simulink model "Assignment_model"  (R2015b)
settings: Solver=ode45  StartTime=0.0  StopTime=50  RelTol=1e-3
settings Model: Creator=Administrator  LastModifiedBy=raghavv
settings DataIOCC: SaveFormat=Array
settings DebuggingCC: SolverPrmCheckMsg=warning
settings HardwareCC: ProdBitPerPointer=32  ProdLargestAtomicFloat=None  ProdIntDivRoundTo=Undefined  ProdEndianess=Unspecified  ProdWordSize=32  ProdHWDeviceType=32-bit Generic
settings GRTTargetCC: GeneratePreprocessorConditionals=Disable all
settings ConfigComp: CovModelRefEnable=Off  CovSFcnEnable=off

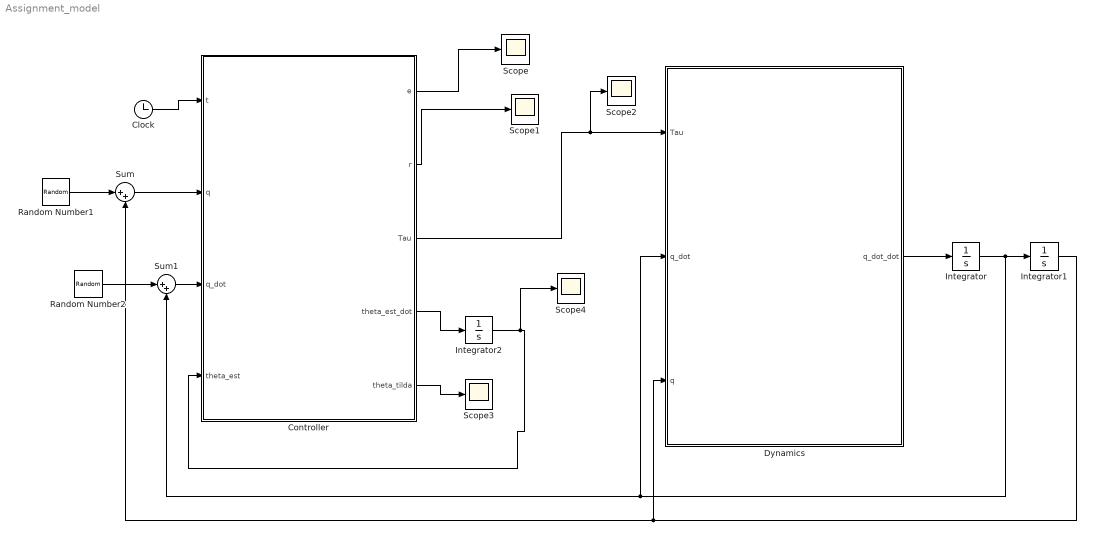
== system Assignment_model ==
  Clock : Clock
      settings: Decimation=50
  Controller : MATLAB Function  TreatAsAtomicUnit=on
  Dynamics : MATLAB Function  TreatAsAtomicUnit=on
  Integrator : Integrator  InitialCondition=[1;-1]
  Integrator1 : Integrator  InitialCondition=[1,1]
  Integrator2 : Integrator  InitialCondition=rand(5,1)
  Random Number1 : RandomNumber  Variance=0  SampleTime=0.1
  Random Number2 : RandomNumber  Variance=0  SampleTime=0.1
  Scope{,1..4} (5 alike) : Scope
  Sum : Sum  Inputs=|++
  Sum1 : Sum  Inputs=|++
  wires:
  Dynamics/1(q_dot_dot) -> Integrator/1
  Integrator/1 -> Sum1/2, Dynamics/2(q_dot), Integrator1/1
  Integrator1/1 -> Sum/2, Dynamics/3(q)
  Controller/3(Tau) -> Scope2/1, Dynamics/1(Tau)
  Clock/1 -> Controller/1(t)
  Controller/1(e) -> Scope/1
  Controller/2(r) -> Scope1/1
  Controller/4(theta_est_dot) -> Integrator2/1
  Integrator2/1 -> Scope4/1, Controller/4(theta_est)
  Controller/5(theta_tilda) -> Scope3/1
  Random Number2/1 -> Sum1/1
  Random Number1/1 -> Sum/1
  Sum/1 -> Controller/2(q)
  Sum1/1 -> Controller/3(q_dot)

== matlab function Assignment_model/Controller ==
  data: e output; r output; Tau output; t input; q input; q_dot input; theta_est input; theta_est_dot output; theta_tilda output
function [e,r,Tau, theta_est_dot, theta_tilda] = controller(t,q,q_dot,theta_est)
%Raghavv Goel | 2016179
c2=cos(q(2));
s2=sin(q(2));
alpha=10;
k=10;

p1=3.473;
p2=0.196;
p3=0.242;
fd1=5.3;
fd2=1.1;

theta = [p1;p2;p3;fd1;fd2];

qd=[0.5*sin(t);2*cos(t/4)];
qd_dot=[0.5*cos(t);-0.5*sin(t/4)];
qd_ddot=[-0.5*sin(t);-0.25*cos(t/4)];
e=q-qd;     %Tracking Error
e_dot=q_dot-qd_dot;

r=e_dot+alpha*e;         %Filtered Tracking Error

y = 10*eye(5);
%----------------------------------------------------------%
%M=[p1+2*p3*c2 p2+p3*c2;p2+p3*c2 p2];% Inertia matrix
%Vm=[-p3*s2*q_dot(2) -p3*s2*(q_dot(1)+q_dot(2));p3*s2*q_dot(1) 0];%Centripetal coriolis matrix
%fd=[fd1 0;0 fd2]; % Friction matrix

z1 = [-qd_ddot(1) + alpha*e_dot(1) ; 0];
z2 = [-qd_ddot(2) + alpha*e_dot(2) ; -qd_ddot(1) -  qd_ddot(2) + alpha*(e_dot(1) + e_dot(2))];
z3 = [2*c2*(-qd_ddot(1) + alpha*e_dot(1)) + c2*(-qd_ddot(2) + alpha*e_dot(2)) + s2*q_dot(2)*(q_dot(1) + r(1)) + s2*(q_dot(1) + q_dot(2))*(q_dot(2) + r(2)) ;
      c2*(-qd_ddot(1) + alpha*e_dot(1)) - s2*q(1)*(q_dot(1) + r(1))  ];
z4 = [-q_dot(1); 0];
z5 = [0; -q_dot(2)];

Z = [z1 z2 z3 z4 z5];
%Z = [-qd_ddot(1) + alpha*q_dot(1) - alpha*qd_dot(1), -qd_ddot(2) + alpha*(q_dot(2) - qd_dot(2)), -2*c2*qd_ddot(1) - c2*qd_ddot(2) + 2*s2*q_dot(1)*q_dot(2) + s2*q_dot(2)*q_dot(2) + 2*alpha*c2*(q_dot(1) - qd_dot(1)) + alpha*c2*(q_dot(2) - qd_dot(2)), q_dot(1) , 0 ; 0, -qd_ddot(1) - qd_ddot(2) + alpha*(q_dot(1) + q_dot(2) - qd_dot(1) - qd_dot(2)),  -c2*qd_ddot(1) - s2*q_dot(1)*q_dot(1) + alpha*(q_dot(1) - qd_dot(1)), 0, q_dot(2)];

theta_est_dot = y*Z'*r;

Tau = -Z*theta_est - k*r - e;
%tau=-k*r+Vm*q_dot+fd*q_dot+M*qd_ddot-alpha*M*e_dot-Vm*r-e;         % Controller
theta_tilda = theta - theta_est;

== matlab function Assignment_model/Dynamics ==
  data: Tau input; q_dot_dot output; q_dot input; q input
function q_dot_dot   = dynamics(Tau,q_dot,q)
%Raghavv Goel | 2016179
%#codegen
p1= 3.473;
p2=0.196;
p3=0.242;
fd1=5.3;
fd2=1.1;

c2=cos(q(2));
s2=sin(q(2));
% alpha=1;
%y = eye(5);

M=[p1+2*p3*c2 p2+p3*c2;p2+p3*c2 p2];% Inertia matrix
Vm=[-p3*s2*q_dot(2) -p3*s2*(q_dot(1)+q_dot(2));p3*s2*q_dot(1) 0];%Centripetal coriolis matrix
fd=[fd1 0;0 fd2]; % Friction matrix
%new dynamics are Z*theta, we have an estimate of theta: theta_est
q_dot_dot=-M\(Vm*q_dot+fd*q_dot-Tau);   %EL dynamics
